simulink model "test_saturation_simulink"  (R2022a)
settings: Solver=VariableStepAuto  StartTime=0.0  StopTime=stop_time  RelTol=1e-3
undefined symbols (not defined in the file or in its folder): amp, amplitude, max_v, min_v, saturation, start_value, ts
libraries: simulink x1
settings Model: Creator=Niccolò  LastModifiedBy=Niccolò

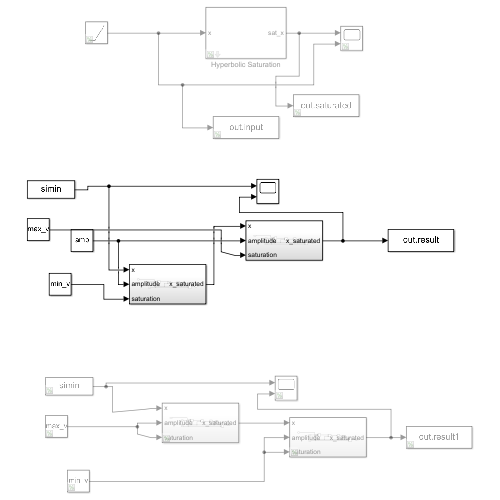
[thumbnail: Simulink's stored preview of the top-level diagram]
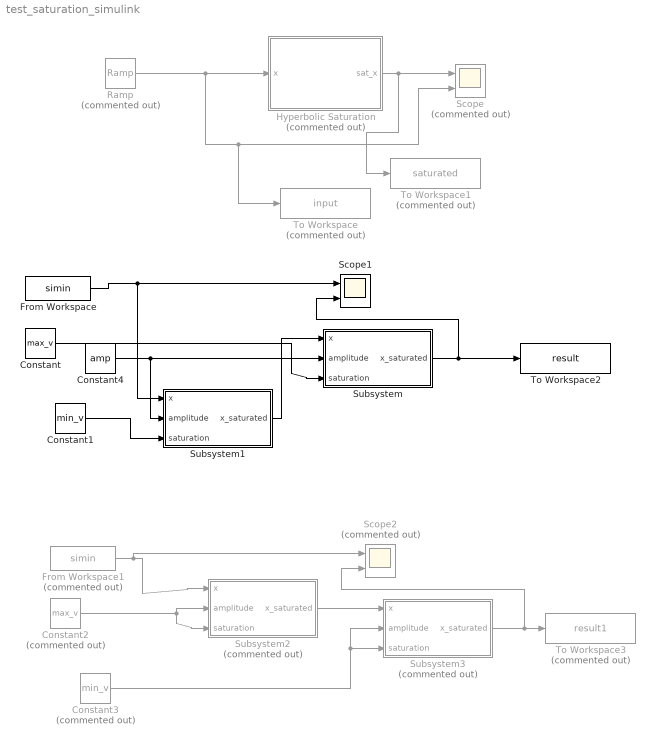
== system test_saturation_simulink ==
  Constant : Constant  Value=max_v
  Constant1 : Constant  Value=min_v
  Constant2 : Constant  Commented=on  Value=max_v
  Constant3 : Constant  Commented=on  Value=min_v
  Constant4 : Constant  Value=amp
  From Workspace : FromWorkspace  VariableName=simin  SampleTime=ts
  From Workspace1 : FromWorkspace  Commented=on  VariableName=simin  SampleTime=ts
  Hyperbolic Saturation : Subsystem  Commented=on  mask{amplitude=amplitude, saturation=saturation}
  Ramp : simulink/Sources/Ramp  Commented=on  slope=1  start=0  InitialOutput=start_value
  Scope : Scope  Commented=on  NumInputPorts=2
  Scope1 : Scope  NumInputPorts=2
  Scope2 : Scope  Commented=on  NumInputPorts=2
  Subsystem : Subsystem
  Subsystem1 : Subsystem
  Subsystem2 : Subsystem  Commented=on
  Subsystem3 : Subsystem  Commented=on
  To Workspace : ToWorkspace  Commented=on  VariableName=input  SaveFormat=Timeseries  SampleTime=-1
  To Workspace1 : ToWorkspace  Commented=on  VariableName=saturated  SaveFormat=Timeseries  SampleTime=-1
  To Workspace2 : ToWorkspace  VariableName=result  SaveFormat=Timeseries  SampleTime=-1
  To Workspace3 : ToWorkspace  Commented=on  VariableName=result1  SaveFormat=Timeseries  SampleTime=-1
  wires:
  Hyperbolic Saturation/1(sat_x) -> To Workspace1/1, Scope/1
  Ramp/1 -> To Workspace/1, Scope/2, Hyperbolic Saturation/1(x)
  From Workspace/1 -> Subsystem1/1(x), Scope1/1
  Constant/1 -> Subsystem/3(saturation)
  Constant1/1 -> Subsystem1/3(saturation)
  From Workspace1/1 -> Scope2/1, Subsystem2/1(x)
  Constant3/1 -> Subsystem3/3(saturation), Subsystem3/2(amplitude)
  Subsystem2/1(x_saturated) -> Subsystem3/1(x)
  Subsystem3/1(x_saturated) -> Scope2/2, To Workspace3/1
  Constant2/1 -> Subsystem2/2(amplitude), Subsystem2/3(saturation)
  Subsystem1/1(x_saturated) -> Subsystem/1(x)
  Subsystem/1(x_saturated) -> Scope1/2, To Workspace2/1
  Constant4/1 -> Subsystem1/2(amplitude), Subsystem/2(amplitude)

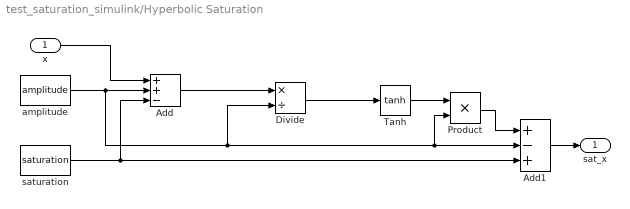
== system test_saturation_simulink/Hyperbolic Saturation ==
  x : Inport
  Add : Sum  Inputs=++-
  Add1 : Sum  Inputs=+-+
  Divide : Product  Inputs=*/
  Product : Product
  Tanh : Trigonometry  Operator=tanh
  amplitude : Constant  Value=amplitude
  saturation : Constant  Value=saturation
  sat_x : Outport
  wires:
  saturation/1 -> Add/3, Add1/3
  Add/1 -> Divide/1
  amplitude/1 -> Divide/2, Product/2, Add1/2, Add/2
  Divide/1 -> Tanh/1
  Add1/1 -> sat_x/1
  Product/1 -> Add1/1
  Tanh/1 -> Product/1
  x/1 -> Add/1

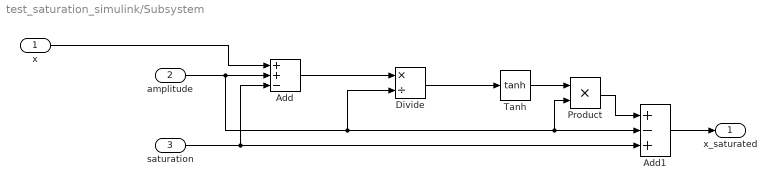
== system test_saturation_simulink/Subsystem ==
  x : Inport
  amplitude : Inport  Port=2
  saturation : Inport  Port=3
  Add : Sum  Inputs=++-
  Add1 : Sum  Inputs=+-+
  Divide : Product  Inputs=*/
  Product : Product
  Tanh : Trigonometry  Operator=tanh
  x_saturated : Outport
  wires:
  saturation/1 -> Add/3, Add1/3
  Product/1 -> Add1/1
  amplitude/1 -> Divide/2, Product/2, Add1/2, Add/2
  Divide/1 -> Tanh/1
  Add/1 -> Divide/1
  Tanh/1 -> Product/1
  Add1/1 -> x_saturated/1
  x/1 -> Add/1

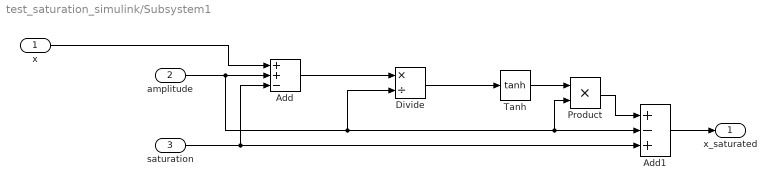
== system test_saturation_simulink/Subsystem1 ==
  x : Inport
  amplitude : Inport  Port=2
  saturation : Inport  Port=3
  Add : Sum  Inputs=++-
  Add1 : Sum  Inputs=+-+
  Divide : Product  Inputs=*/
  Product : Product
  Tanh : Trigonometry  Operator=tanh
  x_saturated : Outport
  wires:
  saturation/1 -> Add/3, Add1/3
  Product/1 -> Add1/1
  amplitude/1 -> Divide/2, Product/2, Add1/2, Add/2
  Divide/1 -> Tanh/1
  Add/1 -> Divide/1
  Tanh/1 -> Product/1
  Add1/1 -> x_saturated/1
  x/1 -> Add/1

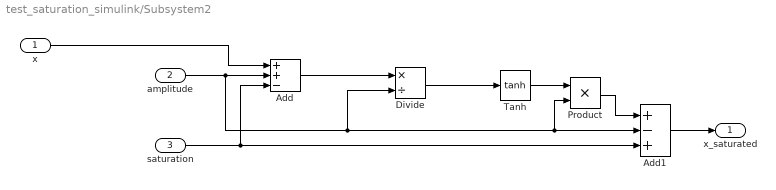
== system test_saturation_simulink/Subsystem2 ==
  x : Inport
  amplitude : Inport  Port=2
  saturation : Inport  Port=3
  Add : Sum  Inputs=++-
  Add1 : Sum  Inputs=+-+
  Divide : Product  Inputs=*/
  Product : Product
  Tanh : Trigonometry  Operator=tanh
  x_saturated : Outport
  wires:
  saturation/1 -> Add/3, Add1/3
  Product/1 -> Add1/1
  amplitude/1 -> Divide/2, Product/2, Add1/2, Add/2
  Divide/1 -> Tanh/1
  Add/1 -> Divide/1
  Tanh/1 -> Product/1
  Add1/1 -> x_saturated/1
  x/1 -> Add/1

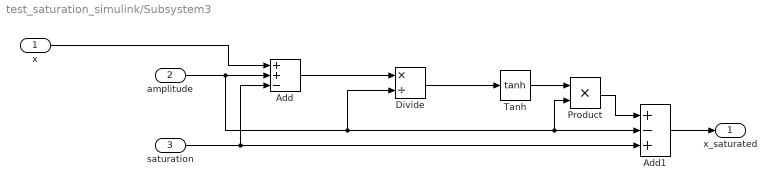
== system test_saturation_simulink/Subsystem3 ==
  x : Inport
  amplitude : Inport  Port=2
  saturation : Inport  Port=3
  Add : Sum  Inputs=++-
  Add1 : Sum  Inputs=+-+
  Divide : Product  Inputs=*/
  Product : Product
  Tanh : Trigonometry  Operator=tanh
  x_saturated : Outport
  wires:
  saturation/1 -> Add/3, Add1/3
  Product/1 -> Add1/1
  amplitude/1 -> Divide/2, Product/2, Add1/2, Add/2
  Divide/1 -> Tanh/1
  Add/1 -> Divide/1
  Tanh/1 -> Product/1
  Add1/1 -> x_saturated/1
  x/1 -> Add/1
